simulink model "verify_Simple_House_SFH15_mdl"  (R2018b)
settings: Solver=ode23tb  StartTime=0  StopTime=365*24*3600  MaxStep=60.0  RelTol=1e-3  EnableMultiTasking=on
undefined symbols (not defined in the file or in its folder): path_carnot
libraries: carnot x5, simulink x3
settings Model: SimulationMode=accelerator  Creator=U_13.adm_zivi  LastModifiedBy=drhf
settings SolverCC: ZeroCrossControl=DisableAll
settings DataIOCC: SaveFormat=Array  SignalLogging=off  DSMLogging=off  ReturnWorkspaceOutputs=on
settings OptimizationCC: LifeSpan=inf  SimCompilerOptimization=on
settings DebuggingCC: ReadBeforeWriteMsg=DisableAll  WriteAfterWriteMsg=DisableAll  WriteAfterReadMsg=DisableAll  UnderspecifiedInitializationDetection=Classic  MergeDetectMultiDrivingBlocksExec=none  SolverPrmCheckMsg=warning  MultiTaskDSMMsg=none  SFUnexpectedBacktrackingDiag=warning  SFNoUnconditionalDefaultTransitionDiag=warning  SFExecutionAtInitializationDiag=none
settings HardwareCC: ProdBitPerPointer=32  ProdBitPerSizeT=32  ProdBitPerPtrDiffT=32  ProdLargestAtomicFloat=None  ProdIntDivRoundTo=Undefined  ProdEndianess=Unspecified  ProdWordSize=32  ProdHWDeviceType=32-bit Generic
settings ModelReferenceCC: UpdateModelReferenceTargets=IfOutOfDate  PropagateSignalLabelsOutOfModel=off
settings SFSimCC: SFSimEcho=off  SimUseLocalCustomCode=off
settings RTWCC: RTWUseLocalCustomCode=off
settings CodeAppCC: StateflowObjectComments=on
settings GRTTargetCC: TargetLangStandard=C89/C90 (ANSI)  GeneratePreprocessorConditionals=Disable all  CombineOutputUpdateFcns=off  GRTInterface=on
settings ConfigComp: CovMetricSettings=dw  CovHtmlReporting=on  CovSaveCumulativeToWorkspaceVar=on  CovSaveSingleToWorkspaceVar=on  CovExternalEMLEnable=off

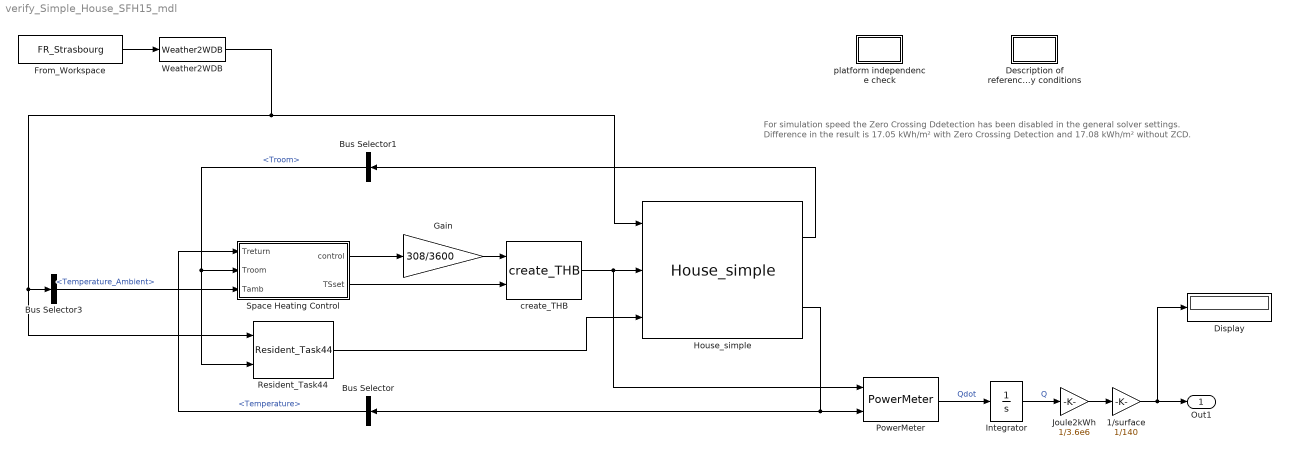
== system verify_Simple_House_SFH15_mdl ==
  note: For simulation speed the Zero Crossing Ddetection has been disabled in the general solver settings.
      | Difference in the result is 17.05 kWh/m² with Zero Crossing Detection and 17.08 kWh/m² without ZCD.
  1/surface : Gain  Gain=1/140
  Bus Selector : BusSelector  OutputSignals=Temperature
  Bus Selector1 : BusSelector  OutputSignals=Troom
  Bus Selector3 : BusSelector  OutputSignals=Temperature_Ambient
  "Description of reference buidling and boundary conditions " : Subsystem
      settings: OpenFcn=|
      | open(fullfile(path_carnot('help'), 'pdf', 'T44A38_Rep_C1_B_ReferenceBuildingDescription_Final_Revised_130906.pdf'));
      | open(fullfile(path_carnot('help'), 'pdf', 'T44A38_Rep_C1_A_BoundaryConditions_Final_Revised_131108.pdf'));
      mask Display: disp('.pdf')
  Display : Display
  From_Workspace : FromWorkspace  VariableName=FR_Strasbourg  SampleTime=0  OutputAfterFinalValue=Setting to zero
  Gain : Gain  Gain=308/3600
  House_simple : carnot/Load/Houses/House_simple  tini=20  dtroom=inf  Tmeaninside=23.8  deltathetai=3.8  Tmeanoutside=11  deltathetae=9.3  tshift=319*3600  PathName=fullfile(path_carnot('libsl'), 'Load', 'Houses', 'House_simple', 'parameter_set')  FileName='SFH15_HouseSimple.mat'  userPath=off  userParam=off  Ahabit=140  Hroom=2.6  slabwidth=10  slablength=7  dwall=0.4  UAwall=0.162*(54.6+26.4)+0.182*((45.7+56.0)*2 -(12+4+3+4))  capa=500000  utot=0.1  gammat=0  cond_ground=2  cp_ground=800  rho_ground=2500  Awindow=[12 4 3 4]  AziWin=[0 90 -180 -90]  Uwindow="[1    1   1    1]*1.0"  Gwindow="[1    1   1    1]*0.585*(1-0.15)"  alpha=10  H=1.2  W=1  Nwin=4  Ventilationrate=0.4  Heatrecovery=0.6  pnom=1792  dtnom=15  expo=1.1  mcap=40000000  lin=10  qua=100
      settings: SourceProductName=Carnot
  Integrator : Integrator
  Joule2kWh : Gain  Gain=1/3.6e6
  PowerMeter : carnot/Control/PowerMeter
      settings: SourceProductName=Carnot
  Resident_Task44 : carnot/Load/Houses/Resident_Task44  period=24*3600  rep_seq_te=[0 1 6 7 8 9 11 12 13 18 19 20 22 23]*3600  rep_seq_de=[1 5 1 1 1 2 1 1 4 2 1 2 1 1]*3600  rep_seq_ye=[105 55 392.5 457.5 420 55 250 55 120 170 615 420 442.5 355]  rep_seq_to=[0 6 7 8 9 11 12 13 14 15 17 18 20 21 22]*3600  rep_seq_do=[6 1 1 1 2 1 1 1 1 2 1 2 1 1 2]*3600  rep_seq_yo=[4 2 3 2 0 1 3 2 1 0 1 2 4 3 4]*60  Topen=24  Tclose=23  TrAboveTa=2  TaTooCold=12  timeFIR=24  TaIni=12  starttime=8  stoptime=22  TroomShadeOn=23.8  TroomShadeOff=22.8  SolarShadeOn=300  SolarShadeOff=200  max_shade=0.25  CalcAirComp=off  mdotCO2=0  mdotH2O=0  mdotVOC=0
      settings: SourceProductName=Carnot
  Space Heating Control : Subsystem  mask{Tset=20, Q_LOC=1792, Td_in=35, Td_out=30, Tambd=-10, n_rad=1.1}
      mask prompts: Tset "desired room Temperature [°C]"; Q_LOC "design heat load [W]"; Td_in "design inlet temperature of the heating system [°C]"; Td_out "design outlet temperature of the heating system [°C]"; Tambd "design outdoor temperature"; n_rad "radiatior exponent"
      mask init:
      | dTd = 0.5*(Td_in + Td_out) - Tset;
  Weather2WDB : carnot/Toolbox/Weather2WDB
      settings: SourceProductName=Carnot
  create_THB : carnot/Source/Simple/create_THB  p=1e5  fluid=Water  mix=0  mix2=0  mix3=0  dia=0.02  hgt=0  mID=No Pressure Drop
      settings: SourceProductName=Carnot
  "platform independence check " : Subsystem
      settings: OpenFcn=open(fullfile(path_carnot('help'), 'pdf', 'Peter_Wintler_Dott_IEA_Task_44_Building_2014.pdf'));
      mask Display: disp('.pdf')
  Out1 : Outport
  wires:
  Space Heating Control/1(control) -> Gain/1
  Weather2WDB/1 -> House_simple/1, Bus Selector3/1, Resident_Task44/1
  create_THB/1 -> PowerMeter/1, House_simple/2
  House_simple/2 -> Bus Selector/1, PowerMeter/2
  Bus Selector/1 -> Space Heating Control/1(Treturn)  "<Temperature>"
  House_simple/1 -> Bus Selector1/1
  Bus Selector3/1 -> Space Heating Control/3(Tamb)  "<Temperature_Ambient>"
  PowerMeter/1 -> Integrator/1  "Qdot"
  1/surface/1 -> Out1/1, Display/1
  Integrator/1 -> Joule2kWh/1  "Q"
  Joule2kWh/1 -> 1/surface/1
  Bus Selector1/1 -> Resident_Task44/2, Space Heating Control/2(Troom)  "<Troom>"
  From_Workspace/1 -> Weather2WDB/1
  Gain/1 -> create_THB/1
  Space Heating Control/2(TSset) -> create_THB/2
  Resident_Task44/1 -> House_simple/3

== system verify_Simple_House_SFH15_mdl/Description of reference buidling and boundary conditions  ==

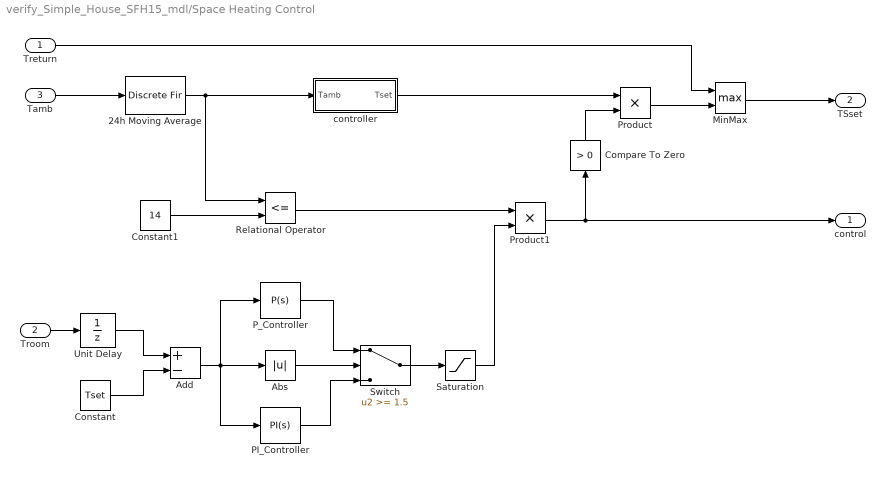
== system verify_Simple_House_SFH15_mdl/Space Heating Control ==
  Treturn : Inport
  Troom : Inport  Port=2
  Tamb : Inport  Port=3
  24h Moving Average : DiscreteFir  Coefficients=ones(1,24)*(1/24)  SampleTime=3600  AccumDataTypeStr=Inherit: Same as product output  RndMeth=Nearest
  Abs : Abs
  Add : Sum  Inputs=+-
  Compare To Zero : simulink/Logic and Bit Operations/Compare To Zero  relop=>  OutDataTypeStr=boolean
  Constant : Constant  Value=Tset
  Constant1 : Constant  Value=14
  MinMax : MinMax  Function=max  Inputs=2
  PI_Controller : simulink/Continuous/PID Controller  Controller=PI  Form=Parallel  TimeDomain=Continuous-time  SampleTime=-1  IntegratorMethod=Forward Euler  FilterMethod=Forward Euler  ControllerParametersSource=internal  P=-0.8  I=-0.05/3600  D=0  UseFilter=on  N=100  TunerSelectOption=Transfer Function Based (PID Tuner App)  ZeroCross=off  InitialConditionSource=internal  InitialConditionForIntegrator=0  InitialConditionForFilter=0  DifferentiatorICPrevScaledInput=0  ExternalReset=none  TrackingMode=off  Kt=1  LimitOutput=on  UpperSaturationLimit=1  LowerSaturationLimit=0  LinearizeAsGain=off  AntiWindupMode=back-calculation  Kb=1  POutMin=[]  POutMax=[]  IOutMin=[]  IOutMax=[]  DOutMin=[]  DOutMax=[]  NOutMin=[]  NOutMax=[]  SumOutMin=[]  SumOutMax=[]  SaturationOutMin=[]  SaturationOutMax=[]  PParamMin=[]  PParamMax=[]  IParamMin=[]  IParamMax=[]  DParamMin=[]  DParamMax=[]  NParamMin=[]  NParamMax=[]  KbParamMin=[]  KbParamMax=[]  KtParamMin=[]  KtParamMax=[]  KbOutMin=[]  KbOutMax=[]  KtOutMin=[]  KtOutMax=[]  IntegratorOutMin=[]  IntegratorOutMax=[]  FilterOutMin=[]  FilterOutMax=[]  SumI1OutMin=[]  SumI1OutMax=[]  SumI2OutMin=[]  SumI2OutMax=[]  SumI3OutMin=[]  SumI3OutMax=[]  SumI4OutMin=[]  SumI4OutMax=[]  SumDOutMin=[]  SumDOutMax=[]  DifferentiatorOutMin=[]  DifferentiatorOutMax=[]  FilterDiffOutCoefMin=[]  FilterDiffOutCoefMax=[]  ReciprocalOutMin=[]  ReciprocalOutMax=[]  SumDenOutMin=[]  SumDenOutMax=[]  SumNumOutMin=[]  SumNumOutMax=[]  DivideOutMin=[]  DivideOutMax=[]  IntegratorContinuousStateAttributes=''  IntegratorStateMustResolveToSignalObject=off  IntegratorRTWStateStorageClass=Auto  FilterContinuousStateAttributes=''  FilterStateMustResolveToSignalObject=off  FilterRTWStateStorageClass=Auto  ParallelPVariant=InternalParameters  IdealPVariant=Disabled  IVariant=InternalParameters  DVariant=Disabled  IntegratorVariant=Continuous  SatVariant=Enabled  AWVariant=BackCalculation  PCopyVariant=Disabled  TRVariant=Disabled  FdbkBlocksVariant=Forward  IdealPFdbkVariant=Disabled  SatFdbkVariant=Disabled  DerivativeFilterVariant=Disabled  NVariant=Disabled  NCopyVariant=Disabled_SignalSpec  FilterICVariant=Disabled  IntegratorICVariant=InternalICs  ExternalResetVariant=Disabled  TRSumVariant=Passthrough  SumFdbkVariant=Disabled  SumVariant=Sum_PI
  P_Controller : simulink/Continuous/PID Controller  Controller=P  Form=Parallel  TimeDomain=Continuous-time  SampleTime=-1  IntegratorMethod=Forward Euler  FilterMethod=Forward Euler  ControllerParametersSource=internal  P=-0.5  I=1  D=0  UseFilter=on  N=100  TunerSelectOption=Transfer Function Based (PID Tuner App)  ZeroCross=off  InitialConditionSource=internal  InitialConditionForIntegrator=0  InitialConditionForFilter=0  DifferentiatorICPrevScaledInput=0  ExternalReset=none  TrackingMode=off  Kt=1  LimitOutput=on  UpperSaturationLimit=1  LowerSaturationLimit=0  LinearizeAsGain=off  AntiWindupMode=none  Kb=1  POutMin=[]  POutMax=[]  IOutMin=[]  IOutMax=[]  DOutMin=[]  DOutMax=[]  NOutMin=[]  NOutMax=[]  SumOutMin=[]  SumOutMax=[]  SaturationOutMin=[]  SaturationOutMax=[]  PParamMin=[]  PParamMax=[]  IParamMin=[]  IParamMax=[]  DParamMin=[]  DParamMax=[]  NParamMin=[]  NParamMax=[]  KbParamMin=[]  KbParamMax=[]  KtParamMin=[]  KtParamMax=[]  KbOutMin=[]  KbOutMax=[]  KtOutMin=[]  KtOutMax=[]  IntegratorOutMin=[]  IntegratorOutMax=[]  FilterOutMin=[]  FilterOutMax=[]  SumI1OutMin=[]  SumI1OutMax=[]  SumI2OutMin=[]  SumI2OutMax=[]  SumI3OutMin=[]  SumI3OutMax=[]  SumI4OutMin=[]  SumI4OutMax=[]  SumDOutMin=[]  SumDOutMax=[]  DifferentiatorOutMin=[]  DifferentiatorOutMax=[]  FilterDiffOutCoefMin=[]  FilterDiffOutCoefMax=[]  ReciprocalOutMin=[]  ReciprocalOutMax=[]  SumDenOutMin=[]  SumDenOutMax=[]  SumNumOutMin=[]  SumNumOutMax=[]  DivideOutMin=[]  DivideOutMax=[]  IntegratorContinuousStateAttributes=''  IntegratorStateMustResolveToSignalObject=off  IntegratorRTWStateStorageClass=Auto  FilterContinuousStateAttributes=''  FilterStateMustResolveToSignalObject=off  FilterRTWStateStorageClass=Auto  ParallelPVariant=InternalParameters  IdealPVariant=Disabled  IVariant=Disabled  DVariant=Disabled  IntegratorVariant=Disabled  SatVariant=Enabled  AWVariant=Disabled  PCopyVariant=Disabled  TRVariant=Disabled  FdbkBlocksVariant=Forward  IdealPFdbkVariant=Disabled  SatFdbkVariant=Disabled  DerivativeFilterVariant=Disabled  NVariant=Disabled  NCopyVariant=Disabled_SignalSpec  FilterICVariant=Disabled  IntegratorICVariant=Disabled  ExternalResetVariant=Disabled  TRSumVariant=Passthrough  SumFdbkVariant=Disabled  SumVariant=Passthrough_P
  Product : Product
  Product1 : Product
  Relational Operator : RelationalOperator  Operator=<=  OutDataTypeStr=boolean  RndMeth=Nearest
  Saturation : Saturate  UpperLimit=1  LowerLimit=0  ZeroCross=off
  Switch : Switch  Threshold=1.5
  Unit Delay : UnitDelay  SampleTime=60
  controller : Subsystem
  control : Outport
  TSset : Outport  Port=2
  wires:
  Tamb/1 -> 24h Moving Average/1
  MinMax/1 -> TSset/1
  Troom/1 -> Unit Delay/1
  Constant1/1 -> Relational Operator/2
  Unit Delay/1 -> Add/1
  Constant/1 -> Add/2
  Add/1 -> P_Controller/1, PI_Controller/1, Abs/1
  Abs/1 -> Switch/2
  P_Controller/1 -> Switch/1
  PI_Controller/1 -> Switch/3
  Switch/1 -> Saturation/1
  Saturation/1 -> Product1/2
  Relational Operator/1 -> Product1/1
  Product/1 -> MinMax/2
  Treturn/1 -> MinMax/1
  Product1/1 -> control/1, Compare To Zero/1
  Compare To Zero/1 -> Product/2
  24h Moving Average/1 -> Relational Operator/1, controller/1(Tamb)
  controller/1(Tset) -> Product/1

== system verify_Simple_House_SFH15_mdl/platform independence check  ==

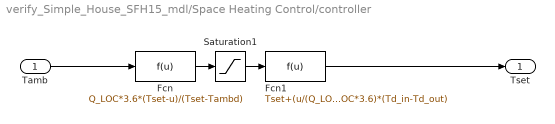
== system verify_Simple_House_SFH15_mdl/Space Heating Control/controller ==
  Tamb : Inport
  Fcn : Fcn  Expr=Q_LOC*3.6*(Tset-u)/(Tset-Tambd)
  Fcn1 : Fcn  Expr=Tset+(u/(Q_LOC*3.6))^(1/n_rad)*dTd+u/(2*Q_LOC*3.6)*(Td_in-Td_out)
  Saturation1 : Saturate  UpperLimit=inf  LowerLimit=0
  Tset : Outport
  wires:
  Tamb/1 -> Fcn/1
  Fcn/1 -> Saturation1/1
  Fcn1/1 -> Tset/1
  Saturation1/1 -> Fcn1/1
